simulink model "plant_lagrangian"  (R2024a)
settings: Solver=VariableStepAuto  StartTime=0.0  StopTime=10.0  FixedStep=0.01  RelTol=1e-3
model mask{considerFem1=1, considerFem2=0, considerFd=0, considerFg=1}
  mask prompts: considerFem1 "Upper inductance"; considerFem2 "Lower inductance"; considerFd "Aerodynamic drag"; considerFg "Gravity"
InitFcn:
  | run("initial_conditions.m")
  | load("parameters_lagrangian.mat")
model workspace (MAT data in the model file):
  considerFd = 0
  considerFem1 = 1
  considerFem2 = 0
  considerFg = 0
undefined symbols (not defined in the file): Cd, g, H, I2min, m, r, R10, R20, rho, v0, x_eq, z0
settings Model: ParameterArgumentNames=considerFd,considerFem1,considerFem2,considerFg  Creator=Bocchio  LastModifiedBy=Bocchio

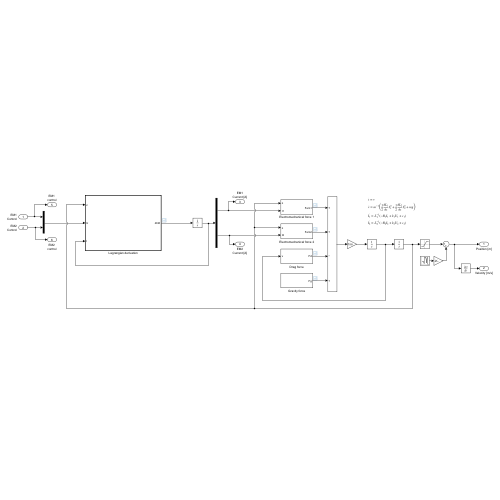
[thumbnail: Simulink's stored preview of the top-level diagram]
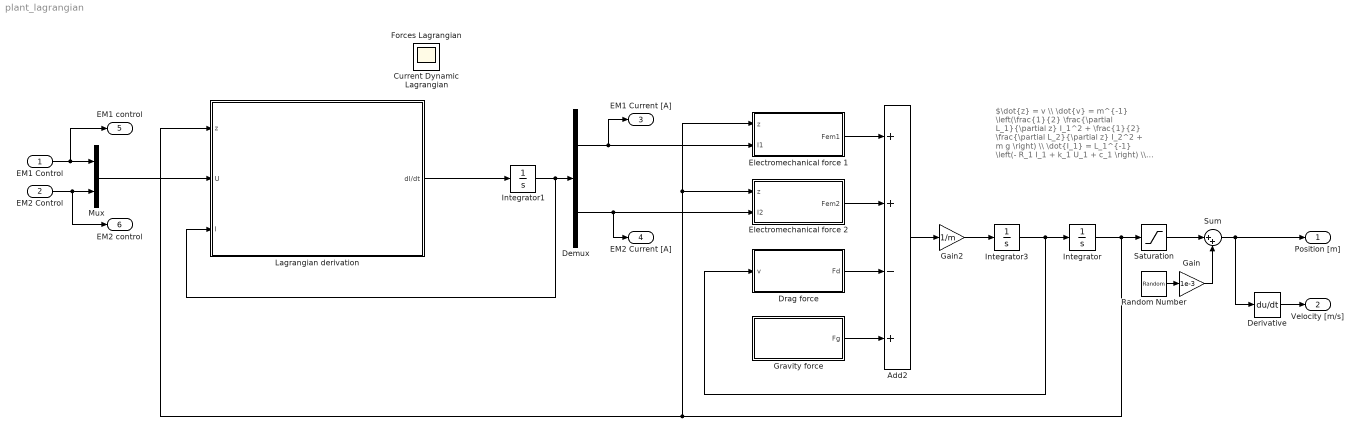
== system plant_lagrangian ==
  note: $\dot{z} = v \\ \dot{v} = m^{-1} \left(\frac{1}{2} \frac{\partial L_1}{\partial z} I_1^2 + \frac{1}{2} \frac{\partial L_2}{\partial z} I_2^2 + m g \right) \\ \dot{I_1} = L_1^{-1} \left(- R_1 I_1 + k_1 U_1 + c_1 \right) \\ \dot{I_2} = L_2^{-1} \left(- R_2 I_2 + k_2 U_2 + c_2 \right)$
  EM1 Control : Inport
  EM2 Control : Inport  Port=2
  Add2 : Sum  Inputs=++-+
  Demux : Demux  Outputs=2
  Derivative : Derivative
  Drag force : Subsystem
  Electromechanical force 1 : Subsystem
  Electromechanical force 2 : Subsystem
  Gain : Gain  Gain=1e-3
  Gain2 : Gain  Gain=1/m
  Gravity force : Subsystem
  Integrator : Integrator  InitialCondition=z0
  Integrator1 : Integrator  InitialCondition=[x_eq(3) I2min]
  Integrator3 : Integrator  InitialCondition=v0
  Lagrangian derivation : Subsystem  TreatAsAtomicUnit=on  VariantControl=currentDynamicModel==2
  Mux : Mux  Inputs=2
  Random Number : RandomNumber  Variance=(1.402804e-3)^2  SampleTime=0.1
  Saturation : Saturate  UpperLimit=H - 2*r  LowerLimit=0
  Sum : Sum  Inputs=|++
  Position [m] : Outport
  Velocity [m/s] : Outport  Port=2
  EM1 Current [A] : Outport  Port=3
  EM2 Current [A] : Outport  Port=4
  EM1 control : Outport  Port=5
  EM2 control : Outport  Port=6
  Current Dynamic Lagrangian : Scope
  Forces Lagrangian : Scope
  wires:
  Integrator/1 -> Saturation/1, Lagrangian derivation/1(z), Electromechanical force 1/1(z), Electromechanical force 2/1(z)
  Add2/1 -> Gain2/1
  Integrator3/1 -> Drag force/1(v), Integrator/1
  EM1 Control/1 -> EM1 control/1, Mux/1
  Gain2/1 -> Integrator3/1
  Demux/1 -> EM1 Current [A]/1, Electromechanical force 1/2(I1)
  Demux/2 -> EM2 Current [A]/1, Electromechanical force 2/2(I2)
  EM2 Control/1 -> EM2 control/1, Mux/2
  Gravity force/1(Fg) -> Add2/4
  Drag force/1(Fd) -> Add2/3
  Electromechanical force 2/1(Fem2) -> Add2/2
  Electromechanical force 1/1(Fem1) -> Add2/1
  Saturation/1 -> Sum/1
  Mux/1 -> Lagrangian derivation/2(U)
  Integrator1/1 -> Lagrangian derivation/3(I), Demux/1
  Lagrangian derivation/1(dI/dt) -> Integrator1/1
  Random Number/1 -> Gain/1
  Sum/1 -> Derivative/1, Position [m]/1
  Derivative/1 -> Velocity [m/s]/1
  Gain/1 -> Sum/2

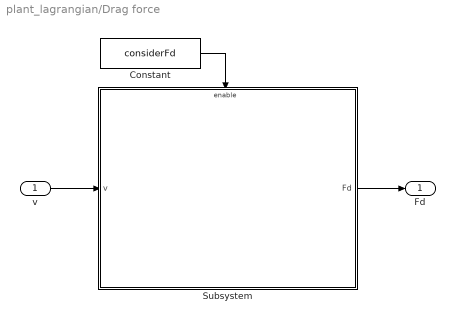
== system plant_lagrangian/Drag force ==
  v : Inport
  Constant : Constant  Value=considerFd
  Subsystem : Subsystem
  Fd : Outport
  wires:
  v/1 -> Subsystem/1(v)
  Subsystem/1(Fd) -> Fd/1
  Constant/1 -> Subsystem/Enable

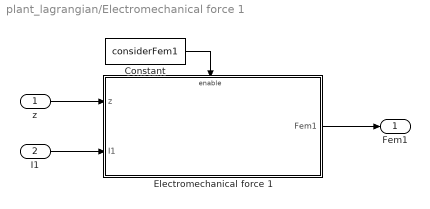
== system plant_lagrangian/Electromechanical force 1 ==
  z : Inport
  I1 : Inport  Port=2
  Constant : Constant  Value=considerFem1
  Electromechanical force 1 : Subsystem  TreatAsAtomicUnit=on
  Fem1 : Outport
  wires:
  z/1 -> Electromechanical force 1/1(z)
  Electromechanical force 1/1(Fem1) -> Fem1/1
  Constant/1 -> Electromechanical force 1/Enable
  I1/1 -> Electromechanical force 1/2(I1)

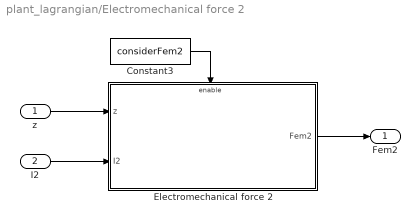
== system plant_lagrangian/Electromechanical force 2 ==
  z : Inport
  I2 : Inport  Port=2
  Constant3 : Constant  Value=considerFem2
  Electromechanical force 2 : Subsystem  TreatAsAtomicUnit=on
  Fem2 : Outport
  wires:
  Constant3/1 -> Electromechanical force 2/Enable
  Electromechanical force 2/1(Fem2) -> Fem2/1
  z/1 -> Electromechanical force 2/1(z)
  I2/1 -> Electromechanical force 2/2(I2)

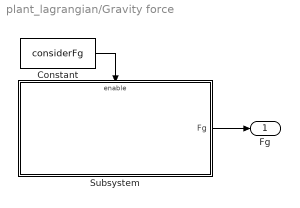
== system plant_lagrangian/Gravity force ==
  Constant : Constant  Value=considerFg
  Subsystem : Subsystem
  Fg : Outport
  wires:
  Subsystem/1(Fg) -> Fg/1
  Constant/1 -> Subsystem/Enable

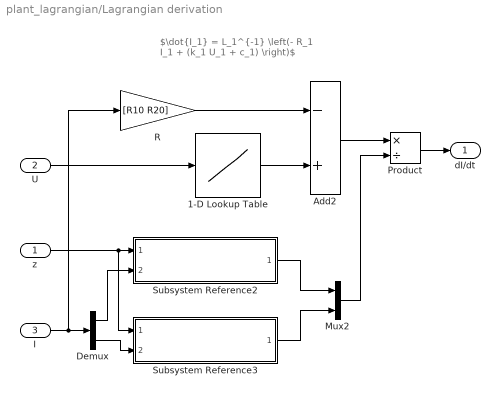
== system plant_lagrangian/Lagrangian derivation ==
  note: $\dot{I_1} = L_1^{-1} \left(- R_1 I_1 + (k_1 U_1 + c_1) \right)$
  z : Inport
  U : Inport  Port=2
  I : Inport  Port=3
  1-D Lookup Table : Lookup_n-D  NumberOfTableDimensions=1  BreakpointsForDimension1=[0 0.05179 1]  Table=[0.0430 0.0430 11.0972]  InternalRulePriority=Speed  RndMeth=Simplest
  Add2 : Sum  Inputs=-+
  Demux : Demux  Outputs=2
  Mux2 : Mux  Inputs=2
  Product : Product  Inputs=*/
  R : Gain  Gain=[R10 R20]
  Subsystem Reference2 : Subsystem  ReferencedSubsystem=L1
  Subsystem Reference3 : Subsystem  ReferencedSubsystem=L2
  dI/dt : Outport
  wires:
  Product/1 -> dI/dt/1
  z/1 -> Subsystem Reference3/1, Subsystem Reference2/1
  Subsystem Reference2/1 -> Mux2/1
  Subsystem Reference3/1 -> Mux2/2
  I/1 -> Demux/1, R/1
  Add2/1 -> Product/1
  R/1 -> Add2/1
  1-D Lookup Table/1 -> Add2/2
  U/1 -> 1-D Lookup Table/1
  Demux/1 -> Subsystem Reference2/2
  Demux/2 -> Subsystem Reference3/2
  Mux2/1 -> Product/2

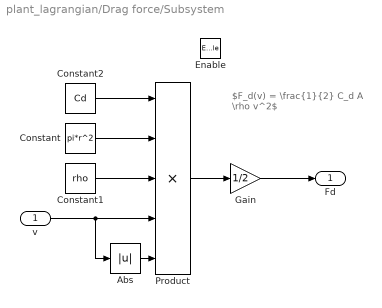
== system plant_lagrangian/Drag force/Subsystem ==
  note: $F_d(v) = \frac{1}{2} C_d A \rho v^2$
  v : Inport
  Enable : EnablePort
  Abs : Abs  SaturateOnIntegerOverflow=off
  Constant : Constant  Value=pi*r^2
  Constant1 : Constant  Value=rho
  Constant2 : Constant  Value=Cd
  Gain : Gain  Gain=1/2
  Product : Product  Inputs=5
  Fd : Outport
  wires:
  Constant/1 -> Product/2
  Constant1/1 -> Product/3
  Constant2/1 -> Product/1
  Gain/1 -> Fd/1
  Product/1 -> Gain/1
  v/1 -> Abs/1, Product/4
  Abs/1 -> Product/5

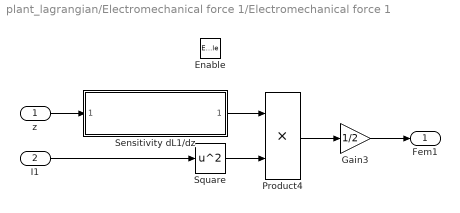
== system plant_lagrangian/Electromechanical force 1/Electromechanical force 1 ==
  z : Inport
  I1 : Inport  Port=2
  Enable : EnablePort
  Gain3 : Gain  Gain=1/2
  Product4 : Product
  Sensitivity dL1/dz : Subsystem  ReferencedSubsystem=dL1dz
  Square : Math  Operator=square
  Fem1 : Outport
  wires:
  I1/1 -> Square/1
  Sensitivity dL1/dz/1 -> Product4/1
  Gain3/1 -> Fem1/1
  z/1 -> Sensitivity dL1/dz/1
  Product4/1 -> Gain3/1
  Square/1 -> Product4/2

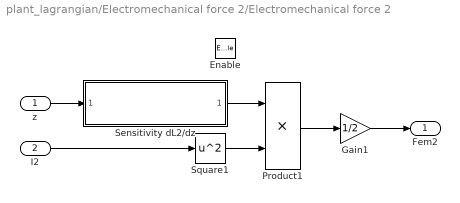
== system plant_lagrangian/Electromechanical force 2/Electromechanical force 2 ==
  z : Inport
  I2 : Inport  Port=2
  Enable : EnablePort
  Gain1 : Gain  Gain=1/2
  Product1 : Product
  Sensitivity dL2/dz : Subsystem  ReferencedSubsystem=dL2dz
  Square1 : Math  Operator=square
  Fem2 : Outport  OutputWhenDisabled=reset  InitialOutput=0
  wires:
  Gain1/1 -> Fem2/1
  Sensitivity dL2/dz/1 -> Product1/1
  I2/1 -> Square1/1
  z/1 -> Sensitivity dL2/dz/1
  Product1/1 -> Gain1/1
  Square1/1 -> Product1/2

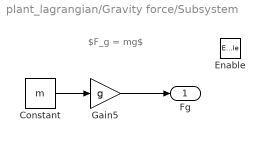
== system plant_lagrangian/Gravity force/Subsystem ==
  note: $F_g = mg$
  Enable : EnablePort
  Constant : Constant  Value=m
  Gain5 : Gain  Gain=g
  Fg : Outport
  wires:
  Gain5/1 -> Fg/1
  Constant/1 -> Gain5/1
